simulink model "MyGearBox_RTW"  (Simulink 10.3)
settings: Solver=ode1  StartTime=0.0  StopTime=inf  FixedStep=0.0002  RelTol=1e-3
PreLoadFcn:
  | vehicle = 'Car'; if ~length(which('cmcmd')), cmenv; end
  | MyGearBox_RTW_bus
InitFcn:
  | vehicle = 'Car'; if ~length(which('cmcmd')), cmenv; end
  | MyGearBox_RTW_bus
undefined symbols (not defined in the file or in its folder): DiscIntNeverNeededParam
libraries: CarMaker4SL x2
Description:
  | CarMaker Plug-in Model Target
settings Model: Creator=ml  ModifiedByFormat=IPG  LastModifiedBy=IPG  MultithreadedSim=on
settings DataIOCC: LimitDataPoints=on
settings DebuggingCC: SFExecutionAtInitializationDiag=warning
settings HardwareCC: TargetHWDeviceType=32-bit Generic  ProdEqTarget=off
settings RTWCC: Description=CarMaker Plug-in Model Target  SystemTargetFile=CarMaker.tlc  TemplateMakefile=CarMaker_unix-win64.tmf
settings CodeAppCC: MaxIdLength=127
settings STFCustomTargetCC: ModelReferenceCompliant=off  CodeInterfacePackaging=Reusable function  CPPClassGenCompliant=on  GRTInterface=off  GenerateAllocFcn=on  SystemTargetFile=CarMaker.tlc
settings GRTTargetCC: ModelReferenceCompliant=off  ParMdlRefBuildCompliant=off  CompOptLevelCompliant=off  ConcurrentExecutionCompliant=off  MatFileLogging=off  CodeInterfacePackaging=Reusable function  GRTInterface=off  GenerateAllocFcn=on  UseToolchainInfoCompliant=off
settings CustomProperty: DataType=string
settings EnumStrPairs: String=Car

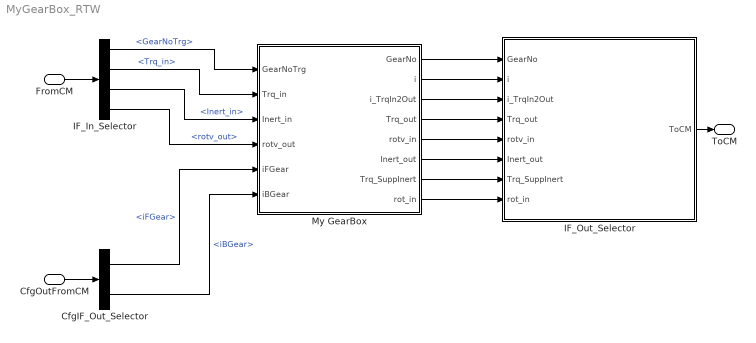
== system MyGearBox_RTW ==
  FromCM : Inport  OutDataTypeStr=Bus: cmPTGearBoxIn
  CfgOutFromCM : Inport  Port=2  OutDataTypeStr=Bus: cmPTGearBoxCfgOut
  CfgIF_Out_Selector : BusSelector  OutputSignals=iFGear,iBGear
  IF_In_Selector : BusSelector  OutputSignals=GearNoTrg,Trq_in,Inert_in,rotv_out
  IF_Out_Selector : Subsystem  mask(Signal Selection){}
      mask help: Signal Selection Block
      settings: OpenFcn=cmSignalSelect('SignalSelection_CB',gcb)
  My GearBox : Subsystem
  ToCM : Outport  OutDataTypeStr=Bus: cmPTGearBoxOut  VectorParamsAs1DForOutWhenUnconnected=off
  wires:
  FromCM/1 -> IF_In_Selector/1
  IF_Out_Selector/1(ToCM) -> ToCM/1
  CfgOutFromCM/1 -> CfgIF_Out_Selector/1
  My GearBox/1(GearNo) -> IF_Out_Selector/1(GearNo)
  My GearBox/2(i) -> IF_Out_Selector/2(i)
  My GearBox/3(i_TrqIn2Out) -> IF_Out_Selector/3(i_TrqIn2Out)
  My GearBox/4(Trq_out) -> IF_Out_Selector/4(Trq_out)
  My GearBox/5(rotv_in) -> IF_Out_Selector/5(rotv_in)
  My GearBox/6(Inert_out) -> IF_Out_Selector/6(Inert_out)
  My GearBox/7(Trq_SuppInert) -> IF_Out_Selector/7(Trq_SuppInert)
  My GearBox/8(rot_in) -> IF_Out_Selector/8(rot_in)
  IF_In_Selector/1 -> My GearBox/1(GearNoTrg)  "<GearNoTrg>"
  IF_In_Selector/2 -> My GearBox/2(Trq_in)  "<Trq_in>"
  IF_In_Selector/3 -> My GearBox/3(Inert_in)  "<Inert_in>"
  IF_In_Selector/4 -> My GearBox/4(rotv_out)  "<rotv_out>"
  CfgIF_Out_Selector/1 -> My GearBox/5(iFGear)  "<iFGear>"
  CfgIF_Out_Selector/2 -> My GearBox/6(iBGear)  "<iBGear>"

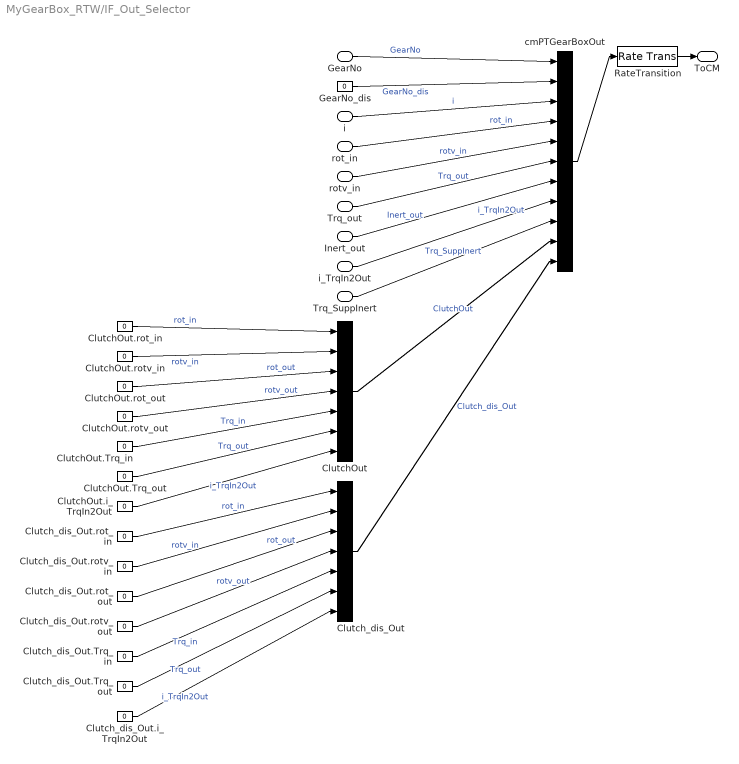
== system MyGearBox_RTW/IF_Out_Selector ==
  GearNo : Inport
  i : Inport  Port=2
  i_TrqIn2Out : Inport  Port=3
  Trq_out : Inport  Port=4
  rotv_in : Inport  Port=5
  Inert_out : Inport  Port=6
  Trq_SuppInert : Inport  Port=7
  rot_in : Inport  Port=8
  ClutchOut : BusCreator  Inputs=7
  ClutchOut.Trq_in : Constant  Value=0
  ClutchOut.Trq_out : Constant  Value=0
  ClutchOut.i_TrqIn2Out : Constant  Value=0
  ClutchOut.rot_in : Constant  Value=0
  ClutchOut.rot_out : Constant  Value=0
  ClutchOut.rotv_in : Constant  Value=0
  ClutchOut.rotv_out : Constant  Value=0
  Clutch_dis_Out : BusCreator  Inputs=7
  Clutch_dis_Out.Trq_in : Constant  Value=0
  Clutch_dis_Out.Trq_out : Constant  Value=0
  Clutch_dis_Out.i_TrqIn2Out : Constant  Value=0
  Clutch_dis_Out.rot_in : Constant  Value=0
  Clutch_dis_Out.rot_out : Constant  Value=0
  Clutch_dis_Out.rotv_in : Constant  Value=0
  Clutch_dis_Out.rotv_out : Constant  Value=0
  GearNo_dis : Constant  Value=0
  RateTransition : RateTransition  OutPortSampleTime=str2num(get_param(bdroot,'FixedStep'))
  cmPTGearBoxOut : BusCreator  Inputs=11
  ToCM : Outport  VectorParamsAs1DForOutWhenUnconnected=off
  wires:
  RateTransition/1 -> ToCM/1
  cmPTGearBoxOut/1 -> RateTransition/1
  GearNo_dis/1 -> cmPTGearBoxOut/2  "GearNo_dis"
  ClutchOut/1 -> cmPTGearBoxOut/10  "ClutchOut"
  ClutchOut.rot_in/1 -> ClutchOut/1  "rot_in"
  ClutchOut.rotv_in/1 -> ClutchOut/2  "rotv_in"
  ClutchOut.rot_out/1 -> ClutchOut/3  "rot_out"
  ClutchOut.rotv_out/1 -> ClutchOut/4  "rotv_out"
  ClutchOut.Trq_in/1 -> ClutchOut/5  "Trq_in"
  ClutchOut.Trq_out/1 -> ClutchOut/6  "Trq_out"
  ClutchOut.i_TrqIn2Out/1 -> ClutchOut/7  "i_TrqIn2Out"
  Clutch_dis_Out/1 -> cmPTGearBoxOut/11  "Clutch_dis_Out"
  Clutch_dis_Out.rot_in/1 -> Clutch_dis_Out/1  "rot_in"
  Clutch_dis_Out.rotv_in/1 -> Clutch_dis_Out/2  "rotv_in"
  Clutch_dis_Out.rot_out/1 -> Clutch_dis_Out/3  "rot_out"
  Clutch_dis_Out.rotv_out/1 -> Clutch_dis_Out/4  "rotv_out"
  Clutch_dis_Out.Trq_in/1 -> Clutch_dis_Out/5  "Trq_in"
  Clutch_dis_Out.Trq_out/1 -> Clutch_dis_Out/6  "Trq_out"
  Clutch_dis_Out.i_TrqIn2Out/1 -> Clutch_dis_Out/7  "i_TrqIn2Out"
  GearNo/1 -> cmPTGearBoxOut/1  "GearNo"
  i/1 -> cmPTGearBoxOut/3  "i"
  i_TrqIn2Out/1 -> cmPTGearBoxOut/8  "i_TrqIn2Out"
  Trq_out/1 -> cmPTGearBoxOut/6  "Trq_out"
  rotv_in/1 -> cmPTGearBoxOut/5  "rotv_in"
  Inert_out/1 -> cmPTGearBoxOut/7  "Inert_out"
  Trq_SuppInert/1 -> cmPTGearBoxOut/9  "Trq_SuppInert"
  rot_in/1 -> cmPTGearBoxOut/4  "rot_in"

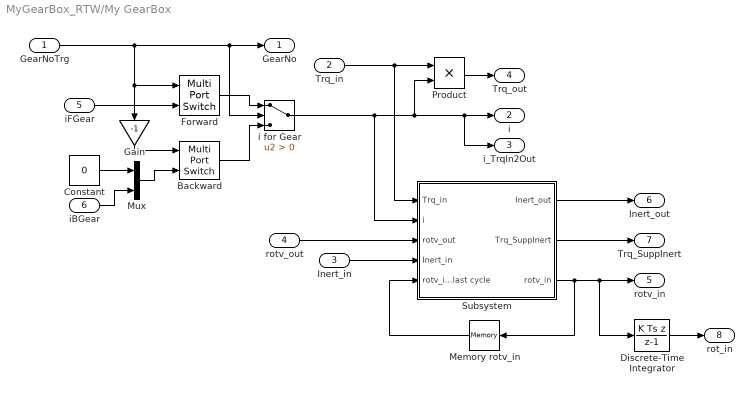
== system MyGearBox_RTW/My GearBox ==
  GearNoTrg : Inport
  Trq_in : Inport  Port=2
  Inert_in : Inport  Port=3
  rotv_out : Inport  Port=4
  iFGear : Inport  Port=5
  iBGear : Inport  Port=6
  Backward : MultiPortSwitch  DataPortOrder=Zero-based contiguous  Inputs=1  zeroidx=on
  Constant : Constant  Value=0
  Discrete-Time Integrator : DiscreteIntegrator  IntegratorMethod=Integration: Backward Euler  SampleTime=-1  ICPrevOutput=DiscIntNeverNeededParam  ICPrevScaledInput=DiscIntNeverNeededParam
  Forward : MultiPortSwitch  Inputs=1
  Gain : Gain  Gain=-1
  Memory rotv_in : Memory
  Mux : Mux  Inputs=2
  Product : Product  RndMeth=Zero
  Subsystem : Subsystem
  i for Gear : Switch  Criteria=u2 > Threshold
  GearNo : Outport  VectorParamsAs1DForOutWhenUnconnected=off
  i : Outport  Port=2  VectorParamsAs1DForOutWhenUnconnected=off
  i_TrqIn2Out : Outport  Port=3  VectorParamsAs1DForOutWhenUnconnected=off
  Trq_out : Outport  Port=4  VectorParamsAs1DForOutWhenUnconnected=off
  rotv_in : Outport  Port=5  VectorParamsAs1DForOutWhenUnconnected=off
  Inert_out : Outport  Port=6  VectorParamsAs1DForOutWhenUnconnected=off
  Trq_SuppInert : Outport  Port=7  VectorParamsAs1DForOutWhenUnconnected=off
  rot_in : Outport  Port=8  VectorParamsAs1DForOutWhenUnconnected=off
  wires:
  GearNoTrg/1 -> i for Gear/2, GearNo/1, Forward/1, Gain/1
  i for Gear/1 -> Product/2, i/1, i_TrqIn2Out/1, Subsystem/2(i)
  Product/1 -> Trq_out/1
  Subsystem/3(rotv_in) -> rotv_in/1, Discrete-Time Integrator/1, Memory rotv_in/1
  Subsystem/1(Inert_out) -> Inert_out/1
  Subsystem/2(Trq_SuppInert) -> Trq_SuppInert/1
  Trq_in/1 -> Product/1, Subsystem/1(Trq_in)
  Forward/1 -> i for Gear/1
  iFGear/1 -> Forward/2
  Backward/1 -> i for Gear/3
  Memory rotv_in/1 -> Subsystem/5(rotv_in last cycle)
  Inert_in/1 -> Subsystem/4(Inert_in)
  rotv_out/1 -> Subsystem/3(rotv_out)
  Gain/1 -> Backward/1
  Discrete-Time Integrator/1 -> rot_in/1
  Mux/1 -> Backward/2
  iBGear/1 -> Mux/2
  Constant/1 -> Mux/1

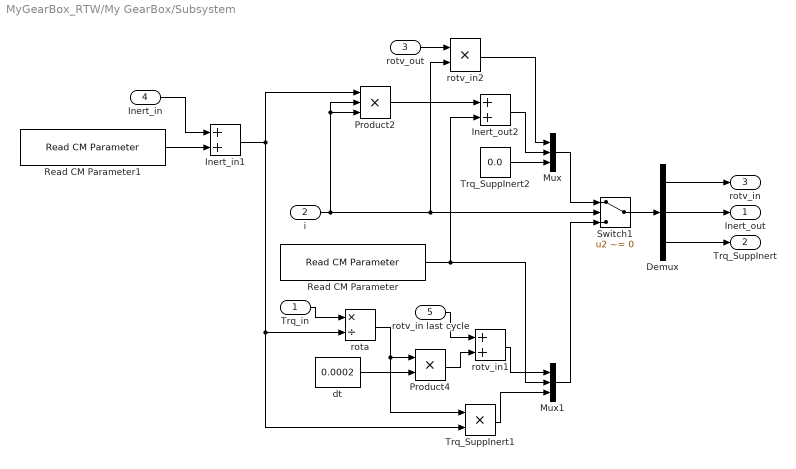
== system MyGearBox_RTW/My GearBox/Subsystem ==
  Trq_in : Inport
  i : Inport  Port=2
  rotv_out : Inport  Port=3
  Inert_in : Inport  Port=4
  rotv_in last cycle : Inport  Port=5
  Demux : Demux  Outputs=3
  Inert_in1 : Sum
  Inert_out2 : Sum
  Mux : Mux  Inputs=3
  Mux1 : Mux  Inputs=3
  Product2 : Product  Inputs=3  RndMeth=Zero
  Product4 : Product  RndMeth=Zero
  Read CM Parameter : CarMaker4SL/Read CM Parameter  xfile=Vehicle  xkey=PowerTrain.GearBox.I_out  xnout=1  xdefaults=0.05  xmuxed=on
      settings: SourceProductName=CarMaker4SL
  Read CM Parameter1 : CarMaker4SL/Read CM Parameter  xfile=Vehicle  xkey=PowerTrain.GearBox.I_in  xnout=1  xdefaults=1e-4  xmuxed=on
      settings: SourceProductName=CarMaker4SL
  Switch1 : Switch  Criteria=u2 ~= 0
  Trq_SuppInert1 : Product  RndMeth=Zero
  Trq_SuppInert2 : Constant  Value=0.0
  dt : Constant  Value=0.0002
  rota : Product  Inputs=*/
  rotv_in1 : Sum
  rotv_in2 : Product  RndMeth=Zero
  Inert_out : Outport  VectorParamsAs1DForOutWhenUnconnected=off
  Trq_SuppInert : Outport  Port=2  VectorParamsAs1DForOutWhenUnconnected=off
  rotv_in : Outport  Port=3  VectorParamsAs1DForOutWhenUnconnected=off
  wires:
  i/1 -> Switch1/2, rotv_in2/2, Product2/2, Product2/3
  Trq_SuppInert2/1 -> Mux/3
  Inert_in/1 -> Inert_in1/1
  Read CM Parameter1/1 -> Inert_in1/2
  rotv_in2/1 -> Mux/1
  Product2/1 -> Inert_out2/1
  Read CM Parameter/1 -> Inert_out2/2, Mux1/2
  Inert_out2/1 -> Mux/2
  Inert_in1/1 -> Product2/1, Trq_SuppInert1/2, rota/2
  Trq_SuppInert1/1 -> Mux1/3
  rota/1 -> Trq_SuppInert1/1, Product4/1
  dt/1 -> Product4/2
  Product4/1 -> rotv_in1/2
  rotv_in1/1 -> Mux1/1
  Demux/1 -> rotv_in/1
  Demux/2 -> Inert_out/1
  Demux/3 -> Trq_SuppInert/1
  Switch1/1 -> Demux/1
  Trq_in/1 -> rota/1
  rotv_in last cycle/1 -> rotv_in1/1
  Mux/1 -> Switch1/1
  Mux1/1 -> Switch1/3
  rotv_out/1 -> rotv_in2/1
